simulink model "PB_skyhook_model"  (R2016b)
settings: Solver=ode23  StartTime=0.0  StopTime=5  RelTol=1e-3
values from neighbouring files (symbols this model uses):
  A = [0                    1              0                0 ... (first row only)    [H_inf_ctrl.m]
  As = [0                   1              0                0 ... (first row only)    [H_inf_ctrl.m]
  B = [0                    0              0                 0 ... (first row only)    [H_inf_ctrl.m]
  Bs = [0                    0              0                 0 ... (first row only)    [H_inf_ctrl.m]
  C = [1, 0, 0, 0 ... (first row only)    [H_inf_ctrl.m]
  Cs = [1, 0, 0, 0 ... (first row only)    [H_inf_ctrl.m]
  cx = 6.32*10^6    (= 6320000)    [H_inf_ctrl.m]
  cz = 1.52*10^5    (= 152000)    [H_inf_ctrl.m]
  D = zeros(2,4)    [H_inf_ctrl.m]
  Ds = zeros(4,4)    [H_inf_ctrl.m]
  f1 = 1    [H_inf_ctrl.m]
  f2 = 8    [H_inf_ctrl.m]
  L1 = 6    [H_inf_ctrl.m]
  L2 = L1    (= 6)    [H_inf_ctrl.m]
undefined symbols (not defined in the file or in its folder): Ainf, Binf, Cinf, Dinf
settings Model: Creator=maxah  LastModifiedBy=maxah

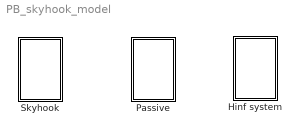
== system PB_skyhook_model ==
  Hinf system : Subsystem
  "Passive " : Subsystem
  Skyhook : Subsystem

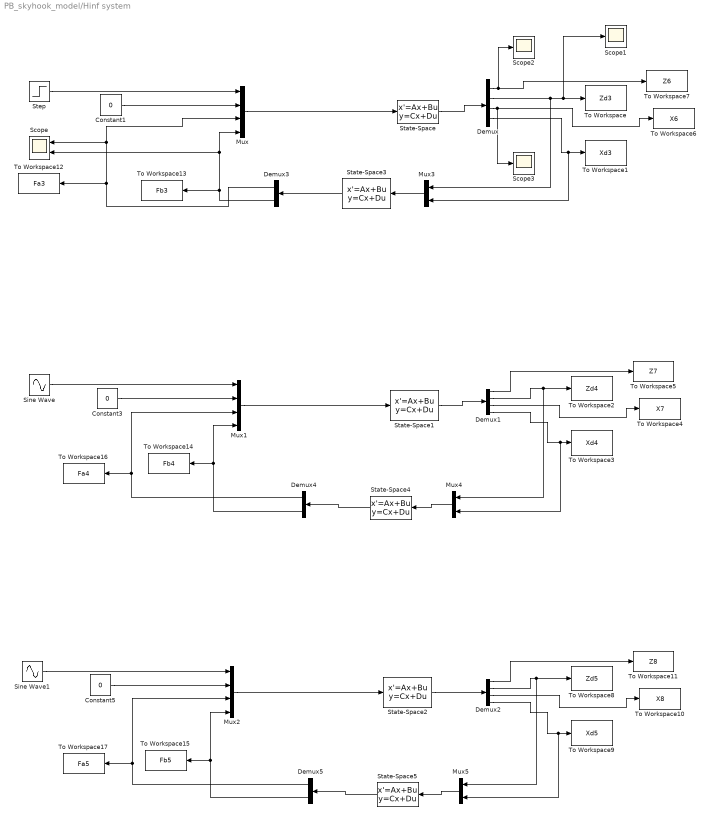
== system PB_skyhook_model/Hinf system ==
  Constant1 : Constant  Value=0
  Constant3 : Constant  Value=0
  Constant5 : Constant  Value=0
  Demux : Demux
  Demux1 : Demux
  Demux2 : Demux
  Demux3 : Demux  Outputs=2
  Demux4 : Demux  Outputs=2
  Demux5 : Demux  Outputs=2
  Mux : Mux
  Mux1 : Mux
  Mux2 : Mux
  Mux3 : Mux  Inputs=2
  Mux4 : Mux  Inputs=2
  Mux5 : Mux  Inputs=2
  Scope : Scope  NumInputPorts=2
  Scope1 : Scope
  Scope2 : Scope
  Scope3 : Scope
  Sine Wave : Sin  Amplitude=0.01  Frequency=2*pi*f1  SampleTime=0
  Sine Wave1 : Sin  Amplitude=0.01  Frequency=2*pi*f2  SampleTime=0
  State-Space : StateSpace  A=As  B=Bs  C=Cs  D=Ds  X0=0
  State-Space1 : StateSpace  A=As  B=Bs  C=Cs  D=Ds  X0=0
  State-Space2 : StateSpace  A=As  B=Bs  C=Cs  D=Ds  X0=0
  State-Space3 : StateSpace  A=Ainf  B=Binf  C=Cinf  D=Dinf  X0=0
  State-Space4 : StateSpace  A=Ainf  B=Binf  C=Cinf  D=Dinf  X0=0
  State-Space5 : StateSpace  A=Ainf  B=Binf  C=Cinf  D=Dinf  X0=0
  Step : Step  After=0.03  SampleTime=0
  To Workspace : ToWorkspace  VariableName=Zd3  SampleTime=-1
  To Workspace1 : ToWorkspace  VariableName=Xd3  SampleTime=-1
  To Workspace10 : ToWorkspace  VariableName=X8  SampleTime=-1
  To Workspace11 : ToWorkspace  VariableName=Z8  SampleTime=-1
  To Workspace12 : ToWorkspace  VariableName=Fa3  SampleTime=-1
  To Workspace13 : ToWorkspace  VariableName=Fb3  SampleTime=-1
  To Workspace14 : ToWorkspace  VariableName=Fb4  SampleTime=-1
  To Workspace15 : ToWorkspace  VariableName=Fb5  SampleTime=-1
  To Workspace16 : ToWorkspace  VariableName=Fa4  SampleTime=-1
  To Workspace17 : ToWorkspace  VariableName=Fa5  SampleTime=-1
  To Workspace2 : ToWorkspace  VariableName=Zd4  SampleTime=-1
  To Workspace3 : ToWorkspace  VariableName=Xd4  SampleTime=-1
  To Workspace4 : ToWorkspace  VariableName=X7  SampleTime=-1
  To Workspace5 : ToWorkspace  VariableName=Z7  SampleTime=-1
  To Workspace6 : ToWorkspace  VariableName=X6  SampleTime=-1
  To Workspace7 : ToWorkspace  VariableName=Z6  SampleTime=-1
  To Workspace8 : ToWorkspace  VariableName=Zd5  SampleTime=-1
  To Workspace9 : ToWorkspace  VariableName=Xd5  SampleTime=-1
  wires:
  Sine Wave/1 -> Mux1/1
  Mux1/1 -> State-Space1/1
  Constant3/1 -> Mux1/2
  Sine Wave1/1 -> Mux2/1
  Mux2/1 -> State-Space2/1
  Constant5/1 -> Mux2/2
  Mux/1 -> State-Space/1
  Step/1 -> Mux/1
  State-Space/1 -> Demux/1
  Constant1/1 -> Mux/2
  Demux2/3 -> To Workspace10/1
  Demux2/2 -> Mux5/1, To Workspace8/1
  Demux/4 -> Mux3/2, To Workspace1/1
  Demux2/4 -> Mux5/2, To Workspace9/1
  Demux1/3 -> To Workspace4/1
  State-Space1/1 -> Demux1/1
  Demux2/1 -> To Workspace11/1
  Demux/1 -> Scope2/1, To Workspace7/1
  Demux/2 -> Mux3/1, Scope1/1, To Workspace/1
  Demux1/2 -> Mux4/1, To Workspace2/1
  Demux1/1 -> To Workspace5/1
  Demux1/4 -> Mux4/2, To Workspace3/1
  Demux/3 -> Scope3/1, To Workspace6/1
  State-Space2/1 -> Demux2/1
  Mux3/1 -> State-Space3/1
  State-Space3/1 -> Demux3/1
  Demux3/1 -> To Workspace12/1, Scope/1, Mux/3
  Demux3/2 -> To Workspace13/1, Scope/2, Mux/4
  Mux4/1 -> State-Space4/1
  State-Space4/1 -> Demux4/1
  Demux4/1 -> To Workspace16/1, Mux1/3
  Demux4/2 -> To Workspace14/1, Mux1/4
  Mux5/1 -> State-Space5/1
  State-Space5/1 -> Demux5/1
  Demux5/1 -> To Workspace17/1, Mux2/3
  Demux5/2 -> To Workspace15/1, Mux2/4

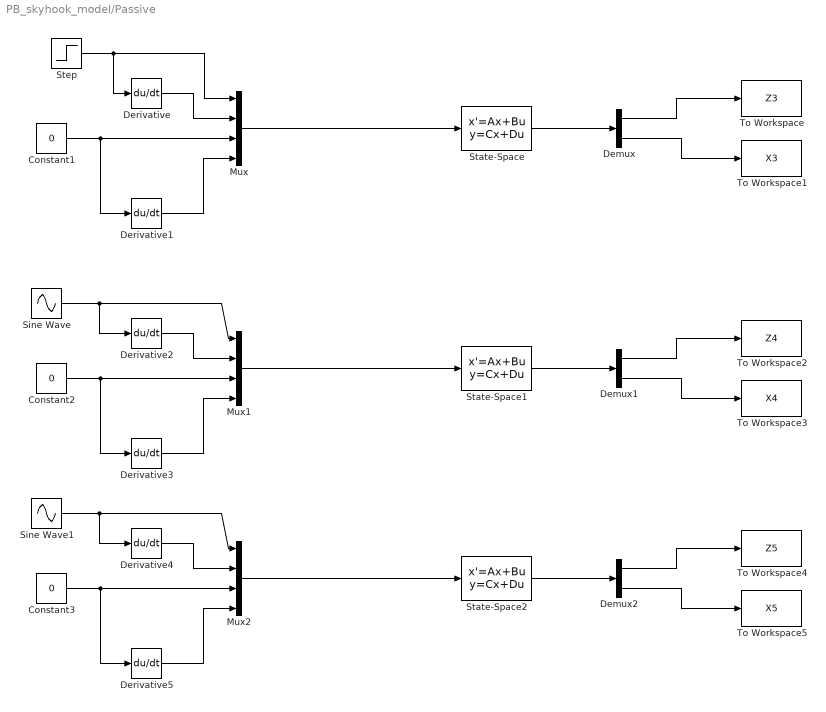
== system PB_skyhook_model/Passive  ==
  Constant1 : Constant  Value=0
  Constant2 : Constant  Value=0
  Constant3 : Constant  Value=0
  Demux : Demux  Outputs=2
  Demux1 : Demux  Outputs=2
  Demux2 : Demux  Outputs=2
  Derivative{,1..5} (6 alike) : Derivative
  Mux : Mux
  Mux1 : Mux
  Mux2 : Mux
  Sine Wave : Sin  Amplitude=0.01  Frequency=2*pi*f1  SampleTime=0
  Sine Wave1 : Sin  Amplitude=0.01  Frequency=2*pi*f2  SampleTime=0
  State-Space : StateSpace  A=A  B=B  C=C  D=D  X0=0
  State-Space1 : StateSpace  A=A  B=B  C=C  D=D  X0=0
  State-Space2 : StateSpace  A=A  B=B  C=C  D=D  X0=0
  Step : Step  After=0.03  SampleTime=0
  To Workspace : ToWorkspace  VariableName=Z3  SampleTime=-1
  To Workspace1 : ToWorkspace  VariableName=X3  SampleTime=-1
  To Workspace2 : ToWorkspace  VariableName=Z4  SampleTime=-1
  To Workspace3 : ToWorkspace  VariableName=X4  SampleTime=-1
  To Workspace4 : ToWorkspace  VariableName=Z5  SampleTime=-1
  To Workspace5 : ToWorkspace  VariableName=X5  SampleTime=-1
  wires:
  Derivative3/1 -> Mux1/4
  Demux1/1 -> To Workspace2/1
  Demux1/2 -> To Workspace3/1
  Sine Wave/1 -> Mux1/1, Derivative2/1
  State-Space1/1 -> Demux1/1
  Mux2/1 -> State-Space2/1
  State-Space2/1 -> Demux2/1
  Demux2/2 -> To Workspace5/1
  Derivative4/1 -> Mux2/2
  Derivative5/1 -> Mux2/4
  Constant3/1 -> Derivative5/1, Mux2/3
  Demux2/1 -> To Workspace4/1
  Sine Wave1/1 -> Derivative4/1, Mux2/1
  Step/1 -> Mux/1, Derivative/1
  Constant1/1 -> Derivative1/1, Mux/3
  Mux/1 -> State-Space/1
  Derivative/1 -> Mux/2
  Derivative1/1 -> Mux/4
  State-Space/1 -> Demux/1
  Demux/2 -> To Workspace1/1
  Constant2/1 -> Mux1/3, Derivative3/1
  Demux/1 -> To Workspace/1
  Mux1/1 -> State-Space1/1
  Derivative2/1 -> Mux1/2

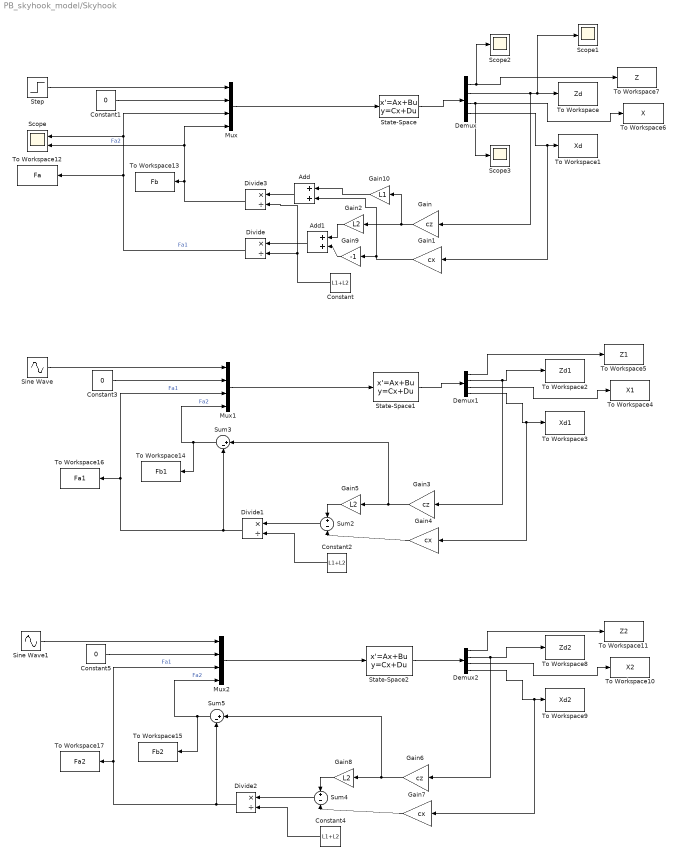
== system PB_skyhook_model/Skyhook ==
  Add : Sum
  Add1 : Sum
  Constant : Constant  Value=L1+L2
  Constant1 : Constant  Value=0
  Constant2 : Constant  Value=L1+L2
  Constant3 : Constant  Value=0
  Constant4 : Constant  Value=L1+L2
  Constant5 : Constant  Value=0
  Demux : Demux
  Demux1 : Demux
  Demux2 : Demux
  Divide{,1..3} (4 alike) : Product  Inputs=*/
  Gain : Gain  Gain=cz
  Gain1 : Gain  Gain=cx
  Gain10 : Gain  Gain=L1
  Gain2 : Gain  Gain=L2
  Gain3 : Gain  Gain=cz
  Gain4 : Gain  Gain=cx
  Gain5 : Gain  Gain=L2
  Gain6 : Gain  Gain=cz
  Gain7 : Gain  Gain=cx
  Gain8 : Gain  Gain=L2
  Gain9 : Gain  Gain=-1
  Mux : Mux
  Mux1 : Mux
  Mux2 : Mux
  Scope : Scope  NumInputPorts=2
  Scope1 : Scope
  Scope2 : Scope
  Scope3 : Scope
  Sine Wave : Sin  Amplitude=0.01  Frequency=2*pi*f1  SampleTime=0
  Sine Wave1 : Sin  Amplitude=0.01  Frequency=2*pi*f2  SampleTime=0
  State-Space : StateSpace  A=As  B=Bs  C=Cs  D=Ds  X0=0
  State-Space1 : StateSpace  A=As  B=Bs  C=Cs  D=Ds  X0=0
  State-Space2 : StateSpace  A=As  B=Bs  C=Cs  D=Ds  X0=0
  Step : Step  After=0.03  SampleTime=0
  Sum2 : Sum  Inputs=+-
  Sum3 : Sum  Inputs=|+-
  Sum4 : Sum  Inputs=+-
  Sum5 : Sum  Inputs=|+-
  To Workspace : ToWorkspace  VariableName=Zd  SampleTime=-1
  To Workspace1 : ToWorkspace  VariableName=Xd  SampleTime=-1
  To Workspace10 : ToWorkspace  VariableName=X2  SampleTime=-1
  To Workspace11 : ToWorkspace  VariableName=Z2  SampleTime=-1
  To Workspace12 : ToWorkspace  VariableName=Fa  SampleTime=-1
  To Workspace13 : ToWorkspace  VariableName=Fb  SampleTime=-1
  To Workspace14 : ToWorkspace  VariableName=Fb1  SampleTime=-1
  To Workspace15 : ToWorkspace  VariableName=Fb2  SampleTime=-1
  To Workspace16 : ToWorkspace  VariableName=Fa1  SampleTime=-1
  To Workspace17 : ToWorkspace  VariableName=Fa2  SampleTime=-1
  To Workspace2 : ToWorkspace  VariableName=Zd1  SampleTime=-1
  To Workspace3 : ToWorkspace  VariableName=Xd1  SampleTime=-1
  To Workspace4 : ToWorkspace  VariableName=X1  SampleTime=-1
  To Workspace5 : ToWorkspace  VariableName=Z1  SampleTime=-1
  To Workspace6 : ToWorkspace  VariableName=X  SampleTime=-1
  To Workspace7 : ToWorkspace  VariableName=Z  SampleTime=-1
  To Workspace8 : ToWorkspace  VariableName=Zd2  SampleTime=-1
  To Workspace9 : ToWorkspace  VariableName=Xd2  SampleTime=-1
  wires:
  Mux1/1 -> State-Space1/1
  Gain5/1 -> Sum2/1
  Gain4/1 -> Sum2/2
  Gain3/1 -> Sum3/1, Gain5/1
  Sum2/1 -> Divide1/1
  Constant2/1 -> Divide1/2
  Divide1/1 -> Sum3/2, To Workspace16/1, Mux1/3  "Fa1"
  Sum3/1 -> To Workspace14/1, Mux1/4  "Fa2"
  Constant3/1 -> Mux1/2
  Sine Wave/1 -> Mux1/1
  Gain6/1 -> Sum5/1, Gain8/1
  Sum4/1 -> Divide2/1
  Constant4/1 -> Divide2/2
  Gain7/1 -> Sum4/2
  Divide2/1 -> Sum5/2, To Workspace17/1, Mux2/3  "Fa1"
  Sum5/1 -> To Workspace15/1, Mux2/4  "Fa2"
  Mux2/1 -> State-Space2/1
  Constant5/1 -> Mux2/2
  Gain8/1 -> Sum4/1
  Sine Wave1/1 -> Mux2/1
  Add1/1 -> Divide/1
  Step/1 -> Mux/1
  State-Space/1 -> Demux/1
  Mux/1 -> State-Space/1
  Gain/1 -> Gain10/1, Gain2/1
  Gain1/1 -> Gain9/1, Add/2
  Gain2/1 -> Add1/1
  Divide3/1 -> Scope/2, Mux/4, To Workspace13/1  "Fa2"
  Constant1/1 -> Mux/2
  Divide/1 -> To Workspace12/1, Mux/3, Scope/1  "Fa1"
  Constant/1 -> Divide3/2, Divide/2
  Demux/4 -> Gain1/1, To Workspace1/1
  Demux2/3 -> To Workspace10/1
  Demux2/2 -> Gain6/1, To Workspace8/1
  Demux2/4 -> Gain7/1, To Workspace9/1
  State-Space2/1 -> Demux2/1
  Demux2/1 -> To Workspace11/1
  Demux/2 -> Gain/1, Scope1/1, To Workspace/1
  Demux1/4 -> Gain4/1, To Workspace3/1
  Demux1/3 -> To Workspace4/1
  State-Space1/1 -> Demux1/1
  Demux1/2 -> Gain3/1, To Workspace2/1
  Demux1/1 -> To Workspace5/1
  Demux/3 -> Scope3/1, To Workspace6/1
  Demux/1 -> Scope2/1, To Workspace7/1
  Gain10/1 -> Add/1
  Add/1 -> Divide3/1
  Gain9/1 -> Add1/2
